simulink model "only_oracle_and_UKF"  (R2019b)
settings: Solver=VariableStepAuto  StartTime=0.0  StopTime=20  RelTol=1e-3
values from neighbouring files (symbols this model uses):
  d = 0.1    [Dynamicfcn.m]    (also in Run_this_file_for_DDWMR_model.m; gps.m)
  I = 0.05    [Dynamicfcn.m]    (also in Run_this_file_for_DDWMR_model.m = 0.26903125)
  L = 0.235/2    (= 0.1175)    [Dynamicfcn.m]    (also in Run_this_file_for_DDWMR_model.m; encoder.m)
  m = 10    [Dynamicfcn.m]    (also in Run_this_file_for_DDWMR_model.m = 15)
  q_initial = [theta_0;x_0;y_0]    [Run_this_file_for_DDWMR_model.m]
  r = 0.05    [Dynamicfcn.m]    (also in Run_this_file_for_DDWMR_model.m; encoder.m; robustness_support.m = temp_r(N+1:-1:1))
  R = 1e-3    (= 0.001)    [Run_this_file_for_DDWMR_model.m]
  Ts = 0.01    [Dynamicfcn.m]    (also in Run_this_file_for_DDWMR_model.m; gps.m = 0.001)
  V_initial = [v_0;w_0]    [Run_this_file_for_DDWMR_model.m]
libraries: simulink x3, sharedTrackingLibrary x1
settings Model: Creator=yu zheng  LastModifiedBy=yu zheng
settings DataIOCC: ReturnWorkspaceOutputsName=out_oracle

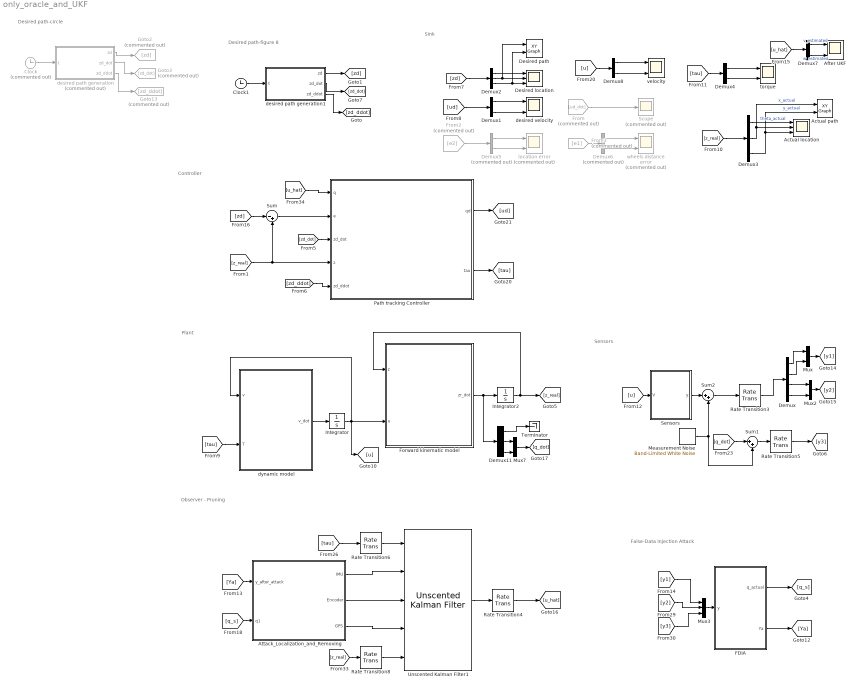
== system only_oracle_and_UKF ==
  note: Plant
  note: Observer - Pruning
  note: Sensors
  note: Controller
  note: Sink
  note: False-Data Injection Attack
  note: Desired path-figure 8
  note: Desired path-circle
  Actual location : Scope  NumInputPorts=3
  Actual path : simulink/Sinks/XY Graph  xmin=-2  xmax=2  ymin=-2  ymax=2  st=-1
  After UKF : Scope  NumInputPorts=2
  Attack_Localization_and_Removing : Subsystem
  Clock : Clock  Commented=on
  Clock1 : Clock
  Demux : Demux
  Demux{1,4,7..8} (4 alike) : Demux  Outputs=2
  Demux11 : Demux  Outputs=3
  Demux2 : Demux  Outputs=3
  Demux3 : Demux  Outputs=3
  Demux5 : Demux  Commented=on  Outputs=2
  Demux6 : Demux  Commented=on  Outputs=2
  Desired location : Scope  NumInputPorts=3
  "Desired path " : simulink/Sinks/XY Graph  xmin=-2  xmax=2  ymin=-2  ymax=2  st=-1
  FDIA : MATLAB Function  TreatAsAtomicUnit=on
  Forward kinematic model : MATLAB Function  TreatAsAtomicUnit=on
  From : From  Commented=on  GotoTag=ud_dot
  From2 : From  Commented=on  GotoTag=e2
  From3 : From  Commented=on  GotoTag=e1
  Goto13 : Goto  Commented=on  GotoTag=zd_ddot
  Goto2 : Goto  Commented=on  GotoTag=zd
  Goto3 : Goto  Commented=on  GotoTag=zd_dot
  Integrator : Integrator  InitialCondition=V_initial
  Integrator2 : Integrator  InitialCondition=q_initial
  Measurement Noise : simulink/Sources/Band-Limited White Noise  Cov=R*Ts  Ts=Ts  seed=[23341]
  Mux : Mux  Inputs=2
  Mux2 : Mux  Inputs=2
  Mux3 : Mux  Inputs=3
  Mux7 : Mux  Inputs=2
  Path tracking Controller : MATLAB Function  TreatAsAtomicUnit=on
  Rate Transition3 : RateTransition  InitialCondition=[0 0 0 0]  OutPortSampleTime=Ts
  Rate Transition4 : RateTransition  Integrity=off  InitialCondition=1.6  OutPortSampleTime=0
  Rate Transition5 : RateTransition  InitialCondition=[0 0 ]  OutPortSampleTime=Ts
  Rate Transition6 : RateTransition  InitialCondition=[0 0]  OutPortSampleTime=Ts
  Rate Transition8 : RateTransition  InitialCondition=[0 0 0]  OutPortSampleTime=Ts
  Scope : Scope  Commented=on
  Sensors : MATLAB Function  TreatAsAtomicUnit=on
  Sum : Sum  Inputs=|-+
  Sum1 : Sum  Inputs=|++
  Sum2 : Sum  Inputs=|++
  Terminator : Terminator
  Unscented Kalman Filter1 : sharedTrackingLibrary/Unscented Kalman Filter  StateTransitionFcn=Dynamicfcn  HasAdditiveProcessNoise=Additive  ProcessNoise=diag([1 1])  HasTimeVaryingProcessNoise=off  HasStateTransitionFcnExtraArgument=1  InitialState=[0 0]  InitialStateCovariance=1e-2  Alpha=1e-2  Beta=2  Kappa=0  MeasurementFcn1=gyroscope  HasMeasurementEnablePort1=off  HasAdditiveMeasurementNoise1=Additive  MeasurementNoise1=diag([R R])  HasTimeVaryingMeasurementNoise1=off  HasMeasurementFcnExtraArgument1=0  MeasurementFcn2=encoder  HasMeasurementEnablePort2=off  HasAdditiveMeasurementNoise2=Additive  MeasurementNoise2=diag([R R])  HasTimeVaryingMeasurementNoise2=off  HasMeasurementFcnExtraArgument2=0  MeasurementFcn3=gps  HasMeasurementEnablePort3=off  HasAdditiveMeasurementNoise3=Additive  MeasurementNoise3=diag([R R])  HasTimeVaryingMeasurementNoise3=off  HasMeasurementFcnExtraArgument3=1  MeasurementFcn4=mfcn3  HasMeasurementEnablePort4=off  HasAdditiveMeasurementNoise4=Additive  MeasurementNoise4=R  HasTimeVaryingMeasurementNoise4=off  HasMeasurementFcnExtraArgument4=0  MeasurementFcn5=myMeasurementFcn  HasMeasurementEnablePort5=off  HasAdditiveMeasurementNoise5=Additive  MeasurementNoise5=1  HasTimeVaryingMeasurementNoise5=off  HasMeasurementFcnExtraArgument5=0  EnableMultirate=off  StateTransitionFcnSampleTime=1  MeasurementFcn1SampleTime=1  MeasurementFcn2SampleTime=1  MeasurementFcn3SampleTime=1  MeasurementFcn4SampleTime=1  MeasurementFcn5SampleTime=1  UseCurrentEstimator=on  OutputStateCovariance=off  DataType=double  SampleTime=Ts  NumberOfMeasurements=3
      settings: SourceProductName=Automated Driving Toolbox  SourceProductBaseCode=DR
  desired path generation : MATLAB Function  Commented=on  TreatAsAtomicUnit=on
  desired path generation1 : MATLAB Function  TreatAsAtomicUnit=on
  desired velocity : Scope  NumInputPorts=2
  dynamic model : MATLAB Function  TreatAsAtomicUnit=on
  location error : Scope  Commented=on  NumInputPorts=2
  torque : Scope  NumInputPorts=2
  velocity : Scope  NumInputPorts=2
  wheels distance error : Scope  Commented=on  NumInputPorts=2
  wires:
  [q_s] -> Attack_Localization_and_Removing/2(q1)
  [Ya] -> Attack_Localization_and_Removing/1(y_after_attack)
  Mux/1 -> [y1]
  Demux/3 -> Mux2/1
  Rate Transition5/1 -> [y3]
  Demux11/2 -> Mux7/1
  Demux4/1 -> torque/1
  [tau] -> Demux4/1
  [ud] -> Demux1/1
  [zd] -> Demux2/1
  Demux6/1 -> wheels distance error/1
  [q_dot] -> Sum1/1
  Demux6/2 -> wheels distance error/2
  [tau] -> dynamic model/2(T)
  Demux2/1 -> Desired location/1
  Demux/4 -> Mux2/2
  Demux1/1 -> desired velocity/1
  From/1 -> Scope/1
  dynamic model/1(v_dot) -> Integrator/1
  [u] -> Sensors/1(V)
  Integrator/1 -> Forward kinematic model/2(u), dynamic model/1(v), [u]
  Integrator2/1 -> [z_real], Forward kinematic model/1(z)
  Demux11/3 -> Mux7/2
  Sum1/1 -> Rate Transition5/1
  Sensors/1(y) -> Sum2/1
  Rate Transition8/1 -> Unscented Kalman Filter1/5
  Demux5/1 -> location error/1
  Mux2/1 -> [y2]
  Demux/2 -> Mux/2
  Attack_Localization_and_Removing/2(Encoder) -> Unscented Kalman Filter1/3
  Unscented Kalman Filter1/1 -> Rate Transition4/1
  Demux2/3 -> "Desired path "/2, Desired location/3
  Rate Transition6/1 -> Unscented Kalman Filter1/1
  Rate Transition3/1 -> Demux/1
  From3/1 -> Demux6/1
  [z_real] -> Rate Transition8/1
  Sum2/1 -> Rate Transition3/1
  From2/1 -> Demux5/1
  Mux7/1 -> [q_dot]
  Demux8/1 -> velocity/1
  [tau] -> Rate Transition6/1
  Demux2/2 -> "Desired path "/1, Desired location/2
  Demux5/2 -> location error/2
  [u] -> Demux8/1
  Rate Transition4/1 -> [u_hat]
  Forward kinematic model/1(zr_dot) -> Demux11/1, Integrator2/1
  Demux8/2 -> velocity/2
  Demux11/1 -> Terminator/1
  Demux/1 -> Mux/1
  Attack_Localization_and_Removing/3(GPS) -> Unscented Kalman Filter1/4
  Measurement Noise/1 -> Sum1/2, Sum2/2
  Demux4/2 -> torque/2
  Demux1/2 -> desired velocity/2
  Attack_Localization_and_Removing/1(IMU) -> Unscented Kalman Filter1/2
  [z_real] -> Demux3/1
  Demux3/3 -> Actual path/2, Actual location/3  "y_actual"
  Demux3/2 -> Actual path/1, Actual location/2  "x_actual"
  Demux3/1 -> Actual location/1  "theta_actual"
  [u_hat] -> Demux7/1
  Demux7/2 -> After UKF/2  "w_estimated"
  Demux7/1 -> After UKF/1  "v_estimated"
  [y3] -> Mux3/3
  Mux3/1 -> FDIA/1(y)
  FDIA/2(Ya) -> [Ya]
  [y1] -> Mux3/1
  FDIA/1(q_actual) -> [q_s]
  [y2] -> Mux3/2
  [u_hat] -> Path tracking Controller/1(q)
  [zd_ddot] -> Path tracking Controller/5(zd_ddot)
  Sum/1 -> Path tracking Controller/2(e)
  [zd_dot] -> Path tracking Controller/3(zd_dot)
  [zd] -> Sum/1
  [z_real] -> Sum/2, Path tracking Controller/4(z)
  Path tracking Controller/1(qd) -> [ud]
  Path tracking Controller/2(tau) -> [tau]
  desired path generation1/1(zd) -> [zd]
  desired path generation1/3(zd_ddot) -> [zd_ddot]
  desired path generation1/2(zd_dot) -> [zd_dot]
  desired path generation/1(zd) -> Goto2/1
  desired path generation/2(zd_dot) -> Goto3/1
  desired path generation/3(zd_ddot) -> Goto13/1
  Clock1/1 -> desired path generation1/1(t)
  Clock/1 -> desired path generation/1(t)

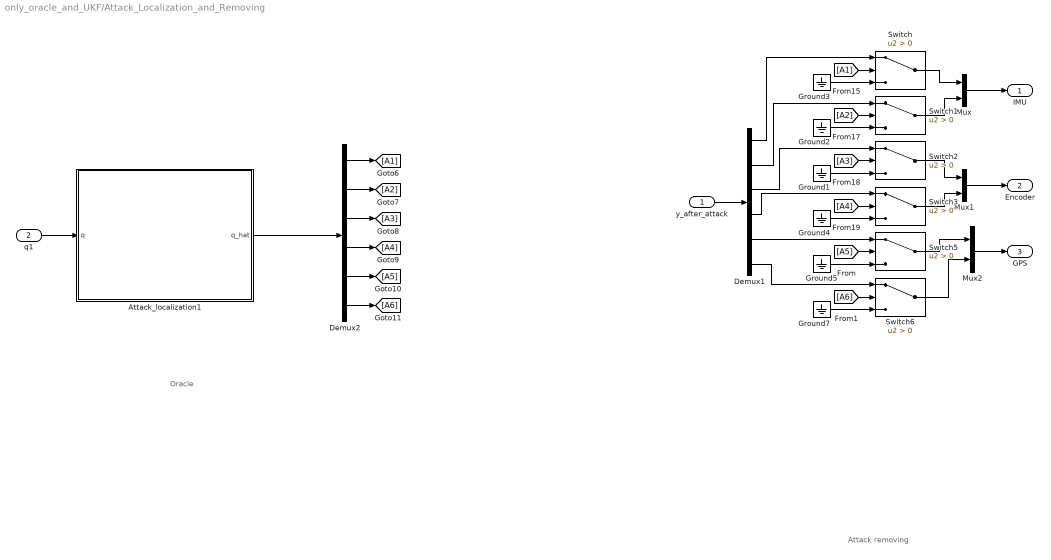
== system only_oracle_and_UKF/Attack_Localization_and_Removing ==
  note: Attack removing
  note: Oracle
  y_after_attack : Inport
  q1 : Inport  Port=2
  Attack_localization1 : MATLAB Function  TreatAsAtomicUnit=on
  Demux1 : Demux  Outputs=6
  Demux2 : Demux  Outputs=6
  Ground{1..5,7} (6 alike) : Ground
  Mux : Mux  Inputs=2
  Mux1 : Mux  Inputs=2
  Mux2 : Mux  Inputs=2
  Switch{,1..3,5..6} (6 alike) : Switch  Criteria=u2 > Threshold
  IMU : Outport
  Encoder : Outport  Port=2
  GPS : Outport  Port=3
  wires:
  [A3] -> Switch2/2
  [A4] -> Switch3/2
  [A2] -> Switch1/2
  [A1] -> Switch/2
  Switch/1 -> Mux/1
  Switch1/1 -> Mux/2
  Switch2/1 -> Mux1/1
  Switch3/1 -> Mux1/2
  Switch6/1 -> Mux2/2
  y_after_attack/1 -> Demux1/1
  Mux/1 -> IMU/1
  Mux2/1 -> GPS/1
  Ground3/1 -> Switch/3
  Demux1/1 -> Switch/1
  Ground2/1 -> Switch1/3
  Ground1/1 -> Switch2/3
  Ground4/1 -> Switch3/3
  Ground5/1 -> Switch5/3
  Ground7/1 -> Switch6/3
  Demux1/2 -> Switch1/1
  Demux1/3 -> Switch2/1
  Demux1/4 -> Switch3/1
  Demux1/5 -> Switch5/1
  Demux1/6 -> Switch6/1
  [A5] -> Switch5/2
  [A6] -> Switch6/2
  Mux1/1 -> Encoder/1
  Switch5/1 -> Mux2/1
  Demux2/3 -> [A3]
  q1/1 -> Attack_localization1/1(q)
  Demux2/2 -> [A2]
  Demux2/6 -> [A6]
  Demux2/1 -> [A1]
  Attack_localization1/1(q_hat) -> Demux2/1
  Demux2/4 -> [A4]
  Demux2/5 -> [A5]

== matlab function only_oracle_and_UKF/Attack_Localization_and_Removing/Attack_localization1 ==
  data: q_hat output; q input; rp parameter
function q_hat  = fcn(q,rp)
%% Obtain oracle

[~, q_hat] = localization_oracle(q,rp);

end

== matlab function only_oracle_and_UKF/FDIA ==
  data: q_actual output; y input; Ya output; d parameter; r parameter; L parameter; Ts parameter; m parameter; I parameter
function [q_actual,Ya] = fcn(y,d,r, L, Ts, m, I)

%% Obtain coding matrix for each time step
theta0=pi/2;
v0=1;
omega0=1;
n  = 3;
T  = 6;    % time horizon (set it equal to number of measurements)

M = diag([m, m*d^2+I]);
D = [0 m*d*omega0;m*d*omega0 0];

C = [                  0,                       1,            0;
                        0,                       0,            1;
                        0,                      1/(4*r),     L/(4*r);
                        0,                      1/(4*r),     -L/(4*r); 
      -v0*sin(theta0)-d*omega0*cos(theta0),  cos(theta0), -d*sin(theta0);
       v0*cos(theta0)+d*omega0*sin(theta0),  sin(theta0),  d*cos(theta0)];
 Cd = C;
 
%  A = [   0,           0,                       1;
%          0,           0,                  2*d*omega0;
%          0,    -m*d*omega0/(m*d^2+I),    -m*d*v0/(m*d^2+I) ];

A = [0 0 1;
     zeros(2,1) -inv(M)*D];

N = size(Cd,1);
Ad = eye(n)+Ts*A;
H = zeros(N*(T+1),n);
%  ya = zeros(N*(T+1),1);
 
 
%% Actual test

% random process to decide the attack nodes
p = 0.8;  % attack (1-p) percentage e.g 20% measurement nodes is attacked
n_safe = fix(p*N); % number of safe measurements
n_attack = N-n_safe; % number of attacked channels

[I_attack_local] = getAttackIndices(Cd,n_attack);

% I_attack = zeros(n_attack*(T+1),1);

% FDIA generation parameters
max_attack = 500;  % maximum allowable attack
tau = .1;   % escape parameter for BDD
I_attack = zeros(n_attack*(T+1),1);
for index=1:(T+1)
    % Building measurement model (linearized)
    H(((index-1)*N+1):(index*N),:) = Cd*Ad^(index-1);  % measurment matrix

    % generating attack indices
%     q = zeros(N,1);
%     q(randperm(N,n_safe)) = 1;
%     I_attack_local = find(~q);  % the attck indices at the current time

    I_attack(((index-1)*n_attack+1):(index*n_attack)) = (index-1)*N + I_attack_local;
        
%     ya(((index-1)*N+1):(index*N),1) = gen_attack_channel(H(((index-1)*size(C,1)+1):(index*size(C,1)),:), max_attack,I_attack,tau);
    
end

ya = gen_attack_channel(H,max_attack,I_attack,tau);

Ya = y+ya(1:N);

q_actual = zeros(6,1);
for ii=1:N
    if ya(ii) == 0
    q_actual(ii) = 1;
    end
end

== matlab function only_oracle_and_UKF/Sensors ==
  data: V input; y output; r parameter; L parameter
function y = fcn(V,r,L)

C=[1,0;
    0,1;
    1/(4*r),L/(4*r);
    1/(4*r),-L/(4*r)];
y=C*V;

== matlab function only_oracle_and_UKF/Path tracking Controller ==
  data: qd output; q input; tau output; e input; zd_dot input; z input; zd_ddot input; m parameter; d parameter; r parameter; L parameter; I parameter
function [qd,tau] = fcn(q,e,zd_dot,z,zd_ddot,m, d, r, L, I)


kq =15;
ke =15;
ez = e(2:3);
% e_theta = e(1);
theta = z(1);
omega = q(2);

B_inver=-(r/(2*L))*[-L,-1;-L,1];
M=[m,0;
    0,m*d*d+I];
D=[0,-m*d*omega;
    m*d*omega,0];
C = [cos(theta), -d*sin(theta);
     sin(theta), d*cos(theta)];
C_bar_tran = [0, cos(theta), sin(theta);
              1, -d*sin(theta), d*cos(theta)];
C_inver = (1/d)*[d*cos(theta), d*sin(theta);
                 -sin(theta), cos(theta)];
C_inver_dot = (1/d)*[-d*sin(theta)*omega, d*cos(theta)*omega;
                     -cos(theta)*omega, -sin(theta)*omega];


qd = C_inver*(zd_dot-ke*ez);
qd_dot = -ke*(C_inver_dot*ez+q)+C_inver*(zd_ddot+ke*zd_dot+C*C_inver_dot*zd_dot);
u = -kq*(q-qd)+qd_dot-C_bar_tran*e;
tau = B_inver*(M*u+D*q);

== matlab function only_oracle_and_UKF/desired path generation1 ==
  data: t input; zd output; zd_dot output; zd_ddot output
function [zd,zd_dot,zd_ddot] = fcn(t)

a=1;
x = a*cos(t)/(1+sin(t)^2);
y = a*sin(t)*cos(t)/(1+sin(t)^2);
% unit circle (radius = 1; origin: (0,0))
zd = [atan(y./x);              % theta
      a*cos(t)/(1+sin(t)^2);         % x
      a*sin(t)*cos(t)/(1+sin(t)^2)];        % y

zd_dot = [-a*sin(t)*(cos(t)^2+2)/(1+sin(t)^2)^2;
          (a*cos(t)^2-2*a*sin(t)^2)/(1+sin(t)^2)^2];

z1 = (a*sin(t)^2*cos(t)^3-11*a*cos(t)^3+8*a*cos(t))/(1+sin(t)^2)^3;
z2 = -2*a*sin(t)*cos(t)*(3+2*cos(t)^2-sin(t)^2)/(1+sin(t)^2)^3;
zd_ddot = [z1;
           z2];

== matlab function only_oracle_and_UKF/Forward kinematic model ==
  data: z input; u input; zr_dot output; d parameter; r parameter
function zr_dot = fcn(z,u,d,r)

%% unpacking the state vectors
theta=z(1);

%% unpacking the intput
v=u(1);
omega=u(2);

%% ODE
theta_dot=omega;
x_dot=v*cos(theta)-d*omega*sin(theta);
y_dot=v*sin(theta)+d*omega*cos(theta);
% phir_dot = (v+omega)/r;
% phil_dot = (v-omega)/r;


%% packing the output
zr_dot=[theta_dot;x_dot;y_dot];

== matlab function only_oracle_and_UKF/dynamic model ==
  data: v_dot output; v input; T input; L parameter; r parameter; d parameter; m parameter; I parameter
function v_dot = fcn(v, T,L, r, d, m,I)

%% unpacking intput
omega=v(2);

%% Parameter
M_temp=[m*d*d+I,0;
         0,m];

M_inver=(1/(m*(m*d*d+I)))*M_temp;

D=[0,-m*d*omega;
    m*d*omega,0];

B=(1/r)*[1,1;L,-L];

%% ODE
v_dot=M_inver*(-D*v+B*T);

== matlab function only_oracle_and_UKF/desired path generation ==
  data: t input; zd output; zd_dot output; zd_ddot output
function [zd,zd_dot,zd_ddot] = fcn(t)


% unit circle (radius = 1; origin: (0,0))
zd = [t;
      cos(t);         % x
      sin(t)];        % y

zd_dot = [-sin(t);
          cos(t)];
      
zd_ddot = [-cos(t);
           -sin(t)];
